simulink model "DSF_CANoe_A3"  (R2022b)
settings: configuration reference "CommonModelConfiguration" (kept outside this file)
undefined symbols (not defined in the file or in its folder): OnOff1, PsdNotPsd
libraries: canoelib x127, simulink x44
(part 2 of 3)

== system DSF_CANoe_A3/ACC//SLA ==
  Constant15 : Constant  Value=0
  Constant17 : Constant  Value=10  OutDataTypeStr=uint8
  Constant18 : Constant  OutDataTypeStr=uint8
  Constant19 : Constant  Value=0  OutDataTypeStr=uint8
  Display44 : Display
  Display48 : Display
  Signal Input3 : canoelib/CANoe I//O/Signal Input  dbName=Backbone  nodeName=DIM  msgName=DIMBackBoneSignalIPdu02  sigName=DrvrCrsCtrlWithBoostReq  editSampleTime=0  rawValue=Default  dataType=Default  dataTypeDB=uint8  hasEncoding=off
      settings: AttributesFormatString=%<sigName>  SourceProductName=Vector CANoe
  Signal Input8 : canoelib/CANoe I//O/Signal Input  dbName=Backbone  nodeName=DIM  msgName=DIMBackBoneSignalIPdu04  sigName=DrvrHmiSpdLimAdpnSts  editSampleTime=0  rawValue=Default  dataType=Default  dataTypeDB=boolean  hasEncoding=off
      settings: AttributesFormatString=%<sigName>  SourceProductName=Vector CANoe
  Signal Output15 : canoelib/CANoe I//O/Signal Output  dbName=Backbone  nodeName=ASDM  msgName=ASDMBackBoneSignalIPdu01  sigName=CnclWarnLatForAutDrv  rawValue=Default  dataType=Default  dataTypeDB=uint8  hasEncoding=off
      settings: AttributesFormatString=%<sigName>  SourceProductName=Vector CANoe
  Signal Output44 : canoelib/CANoe I//O/Signal Output  dbName=Backbone  nodeName=ASDM  msgName=ASDMBackBoneSignalIPdu07  sigName=CtryForRoadSgnInfo  rawValue=Default  dataType=Default  dataTypeDB=uint8  hasEncoding=off
      settings: AttributesFormatString=%<sigName>  SourceProductName=Vector CANoe
  Signal Output45 : canoelib/CANoe I//O/Signal Output  dbName=Backbone  nodeName=IHU  msgName=IHUBackBoneSignalIPdu03  sigName=AccAdprSpdLimActvSts  rawValue=Default  dataType=Default  dataTypeDB=boolean  hasEncoding=off
      settings: AttributesFormatString=%<sigName>  SourceProductName=Vector CANoe
  Signal Output46 : canoelib/CANoe I//O/Signal Output  dbName=Backbone  nodeName=ASDM  msgName=ASDMBackBoneSignalIPdu06  sigName=SpdLimAdpvSts  rawValue=Default  dataType=Default  dataTypeDB=uint8  hasEncoding=off
      settings: AttributesFormatString=%<sigName>  SourceProductName=Vector CANoe
  wires:
  Constant17/1 -> Signal Output44/1
  Constant15/1 -> Signal Output15/1
  Signal Input3/1 -> Display44/1
  Signal Input8/1 -> Display48/1
  Constant18/1 -> Signal Output46/1
  Constant19/1 -> Signal Output45/1

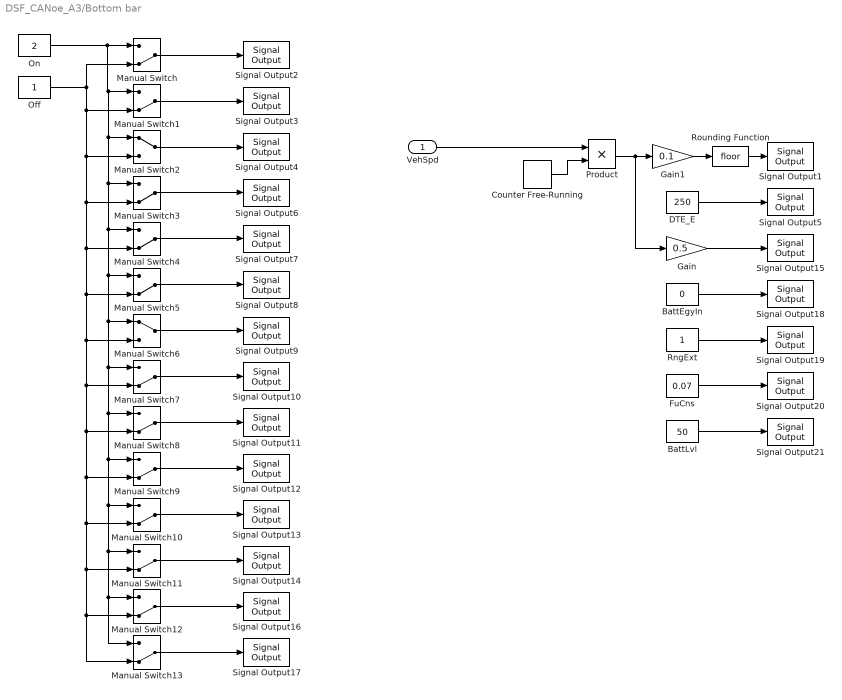
== system DSF_CANoe_A3/Bottom bar ==
  VehSpd : Inport
  BattEgyIn : Constant  Value=0  OutDataTypeStr=uint8
  BattLvl : Constant  Value=50  OutDataTypeStr=uint8
  Counter Free-Running : simulink/Sources/Counter Free-Running  NumBits=8  tsamp=-1
  DTE_E : Constant  Value=250  OutDataTypeStr=uint8
  FuCns : Constant  Value=0.07  OutDataTypeStr=uint8
  Gain : Gain  Gain=0.5
  Gain1 : Gain  Gain=0.1
  Manual Switch{,1,3..5,7..13} (12 alike) : ManualSwitch  CurrentSetting=0
  Manual Switch2 : ManualSwitch
  Manual Switch6 : ManualSwitch
  Off : Constant  OutDataTypeStr=uint8
  On : Constant  Value=2  OutDataTypeStr=uint8
  Product : Product
  RngExt : Constant  OutDataTypeStr=uint8
  Rounding Function : Rounding
  Signal Output1 : canoelib/CANoe I//O/Signal Output  dbName=Backbone  nodeName=VCU1  msgName=VDDMBackBoneSignalIpdu07  sigName=WhlRotCntrFrnt  rawValue=Default  dataType=Default  dataTypeDB=uint8  hasEncoding=off
      settings: AttributesFormatString=%<sigName>  SourceProductName=Vector CANoe
  Signal Output10 : canoelib/CANoe I//O/Signal Output  dbName=Backbone  nodeName=IHU  msgName=IHUBackBoneSignalIPdu07  sigName=SetgAndRstOfTripForDrvrSetgTripForEgyCnsAvg2  rawValue=Default  dataType=Default  dataTypeDB=uint8  hasEncoding=off
      settings: AttributesFormatString=%<sigName>  SourceProductName=Vector CANoe
  Signal Output11 : canoelib/CANoe I//O/Signal Output  dbName=Backbone  nodeName=IHU  msgName=IHUBackBoneSignalIPdu07  sigName=SetgAndRstOfTripForDrvrSetgTripForTiDrv1  rawValue=Default  dataType=Default  dataTypeDB=uint8  hasEncoding=off
      settings: AttributesFormatString=%<sigName>  SourceProductName=Vector CANoe
  Signal Output12 : canoelib/CANoe I//O/Signal Output  dbName=Backbone  nodeName=IHU  msgName=IHUBackBoneSignalIPdu07  sigName=SetgAndRstOfTripForDrvrSetgTripForTiDrv2  rawValue=Default  dataType=Default  dataTypeDB=uint8  hasEncoding=off
      settings: AttributesFormatString=%<sigName>  SourceProductName=Vector CANoe
  Signal Output13 : canoelib/CANoe I//O/Signal Output  dbName=Backbone  nodeName=IHU  msgName=IHUBackBoneSignalIPdu07  sigName=SetgAndRstOfTripForDrvrSetgTripForSpdAvg1  rawValue=Default  dataType=Default  dataTypeDB=uint8  hasEncoding=off
      settings: AttributesFormatString=%<sigName>  SourceProductName=Vector CANoe
  Signal Output14 : canoelib/CANoe I//O/Signal Output  dbName=Backbone  nodeName=IHU  msgName=IHUBackBoneSignalIPdu07  sigName=SetgAndRstOfTripForDrvrSetgTripForSpdAvg2  rawValue=Default  dataType=Default  dataTypeDB=uint8  hasEncoding=off
      settings: AttributesFormatString=%<sigName>  SourceProductName=Vector CANoe
  Signal Output15 : canoelib/CANoe I//O/Signal Output  dbName=Backbone  nodeName=VCU1  msgName=VDDMBackBoneSignalIpdu08  sigName=DispBattEgyOut  rawValue=Default  dataType=Default  dataTypeDB=uint8  hasEncoding=on
      settings: AttributesFormatString=%<sigName>  SourceProductName=Vector CANoe
  Signal Output16 : canoelib/CANoe I//O/Signal Output  dbName=Backbone  nodeName=IHU  msgName=IHUBackBoneSignalIPdu07  sigName=SetgAndRstOfTripForDrvrSetgTripWithProfID  rawValue=Default  dataType=Default  dataTypeDB=uint8  hasEncoding=off
      settings: AttributesFormatString=%<sigName>  SourceProductName=Vector CANoe
  Signal Output17 : canoelib/CANoe I//O/Signal Output  dbName=Backbone  nodeName=CEM  msgName=CEMBackBoneSignalIpdu03  sigName=ProfPenSts1  rawValue=Default  dataType=Default  dataTypeDB=uint8  hasEncoding=off
      settings: AttributesFormatString=%<sigName>  SourceProductName=Vector CANoe
  Signal Output18 : canoelib/CANoe I//O/Signal Output  dbName=Backbone  nodeName=VCU1  msgName=VDDMBackBoneSignalIpdu08  sigName=DispBattEgyIn  rawValue=Default  dataType=Default  dataTypeDB=uint8  hasEncoding=on
      settings: AttributesFormatString=%<sigName>  SourceProductName=Vector CANoe
  Signal Output19 : canoelib/CANoe I//O/Signal Output  dbName=Backbone  nodeName=VCU1  msgName=VDDMBackBoneSignalIpdu08  sigName=RngExtd  rawValue=Default  dataType=Default  dataTypeDB=uint16  hasEncoding=on
      settings: AttributesFormatString=%<sigName>  SourceProductName=Vector CANoe
  Signal Output2 : canoelib/CANoe I//O/Signal Output  dbName=Backbone  nodeName=IHU  msgName=IHUBackBoneSignalIPdu07  sigName=SetgAndRstOfTripForDrvrSetgTripForDstLong  rawValue=Default  dataType=Default  dataTypeDB=uint8  hasEncoding=off
      settings: AttributesFormatString=%<sigName>  SourceProductName=Vector CANoe
  Signal Output20 : canoelib/CANoe I//O/Signal Output  dbName=Backbone  nodeName=VCU1  msgName=VDDMBackBoneSignalIpdu09  sigName=EngFuCnsFild  rawValue=Default  dataType=Default  dataTypeDB=uint8  hasEncoding=on
      settings: AttributesFormatString=%<sigName>  SourceProductName=Vector CANoe
  Signal Output21 : canoelib/CANoe I//O/Signal Output  dbName=Backbone  nodeName=VCU1  msgName=VDDMBackBoneSignalIpdu07  sigName=DispHvBattLvlOfChrg  rawValue=Default  dataType=Default  dataTypeDB=uint16  hasEncoding=on
      settings: AttributesFormatString=%<sigName>  SourceProductName=Vector CANoe
  Signal Output3 : canoelib/CANoe I//O/Signal Output  dbName=Backbone  nodeName=IHU  msgName=IHUBackBoneSignalIPdu07  sigName=SetgAndRstOfTripForDrvrSetgTripForFuCns  rawValue=Default  dataType=Default  dataTypeDB=uint8  hasEncoding=off
      settings: AttributesFormatString=%<sigName>  SourceProductName=Vector CANoe
  Signal Output4 : canoelib/CANoe I//O/Signal Output  dbName=Backbone  nodeName=IHU  msgName=IHUBackBoneSignalIPdu07  sigName=SetgAndRstOfTripForDrvrSetgTripForDstSho1  rawValue=Default  dataType=Default  dataTypeDB=uint8  hasEncoding=off
      settings: AttributesFormatString=%<sigName>  SourceProductName=Vector CANoe
  Signal Output5 : canoelib/CANoe I//O/Signal Output  dbName=Backbone  nodeName=VCU1  msgName=VDDMBackBoneSignalIpdu08  sigName=DstEstimdToEmptyForDrvgElec  rawValue=Default  dataType=Default  dataTypeDB=uint16  hasEncoding=off
      settings: AttributesFormatString=%<sigName>  SourceProductName=Vector CANoe
  Signal Output6 : canoelib/CANoe I//O/Signal Output  dbName=Backbone  nodeName=IHU  msgName=IHUBackBoneSignalIPdu07  sigName=SetgAndRstOfTripForDrvrSetgTripForDstSho2  rawValue=Default  dataType=Default  dataTypeDB=uint8  hasEncoding=off
      settings: AttributesFormatString=%<sigName>  SourceProductName=Vector CANoe
  Signal Output7 : canoelib/CANoe I//O/Signal Output  dbName=Backbone  nodeName=IHU  msgName=IHUBackBoneSignalIPdu07  sigName=SetgAndRstOfTripForDrvrSetgTripForFuCnsAvg1  rawValue=Default  dataType=Default  dataTypeDB=uint8  hasEncoding=off
      settings: AttributesFormatString=%<sigName>  SourceProductName=Vector CANoe
  Signal Output8 : canoelib/CANoe I//O/Signal Output  dbName=Backbone  nodeName=IHU  msgName=IHUBackBoneSignalIPdu07  sigName=SetgAndRstOfTripForDrvrSetgTripForFuCnsAvg2  rawValue=Default  dataType=Default  dataTypeDB=uint8  hasEncoding=off
      settings: AttributesFormatString=%<sigName>  SourceProductName=Vector CANoe
  Signal Output9 : canoelib/CANoe I//O/Signal Output  dbName=Backbone  nodeName=IHU  msgName=IHUBackBoneSignalIPdu07  sigName=SetgAndRstOfTripForDrvrSetgTripForEgyCnsAvg1  rawValue=Default  dataType=Default  dataTypeDB=uint8  hasEncoding=off
      settings: AttributesFormatString=%<sigName>  SourceProductName=Vector CANoe
  wires:
  DTE_E/1 -> Signal Output5/1
  FuCns/1 -> Signal Output20/1
  RngExt/1 -> Signal Output19/1
  Product/1 -> Gain/1, Gain1/1
  BattEgyIn/1 -> Signal Output18/1
  Gain/1 -> Signal Output15/1
  Counter Free-Running/1 -> Product/2
  VehSpd/1 -> Product/1
  Off/1 -> Manual Switch7/2, Manual Switch8/2, Manual Switch9/2, Manual Switch13/2, Manual Switch12/2, Manual Switch11/2, Manual Switch10/2, Manual Switch6/2, Manual Switch5/2, Manual Switch4/2, Manual Switch3/2, Manual Switch2/2, Manual Switch1/2, Manual Switch/2
  Manual Switch/1 -> Signal Output2/1
  On/1 -> Manual Switch2/1, Manual Switch11/1, Manual Switch13/1, Manual Switch12/1, Manual Switch10/1, Manual Switch9/1, Manual Switch8/1, Manual Switch7/1, Manual Switch6/1, Manual Switch5/1, Manual Switch4/1, Manual Switch3/1, Manual Switch1/1, Manual Switch/1
  Manual Switch1/1 -> Signal Output3/1
  Manual Switch2/1 -> Signal Output4/1
  Manual Switch3/1 -> Signal Output6/1
  Manual Switch4/1 -> Signal Output7/1
  Manual Switch5/1 -> Signal Output8/1
  Manual Switch6/1 -> Signal Output9/1
  Manual Switch10/1 -> Signal Output13/1
  Manual Switch13/1 -> Signal Output17/1
  Manual Switch12/1 -> Signal Output16/1
  Manual Switch11/1 -> Signal Output14/1
  Manual Switch9/1 -> Signal Output12/1
  Manual Switch8/1 -> Signal Output11/1
  Manual Switch7/1 -> Signal Output10/1
  BattLvl/1 -> Signal Output21/1
  Gain1/1 -> Rounding Function/1
  Rounding Function/1 -> Signal Output1/1

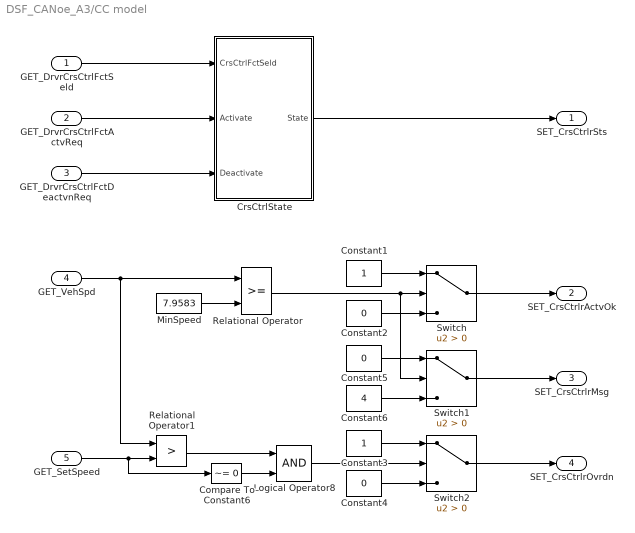
== system DSF_CANoe_A3/CC model ==
  GET_DrvrCrsCtrlFctSeld : Inport
  GET_DrvrCrsCtrlFctActvReq : Inport  Port=2
  GET_DrvrCrsCtrlFctDeactvnReq : Inport  Port=3
  GET_VehSpd : Inport  Port=4
  GET_SetSpeed : Inport  Port=5
  Compare To Constant6 : simulink/Logic and Bit Operations/Compare To Constant  relop=~=  const=0  OutDataTypeStr=boolean
  Constant1 : Constant  OutDataTypeStr=uint8
  Constant2 : Constant  Value=0  OutDataTypeStr=uint8
  Constant3 : Constant  OutDataTypeStr=uint8
  Constant4 : Constant  Value=0  OutDataTypeStr=uint8
  Constant5 : Constant  Value=0  OutDataTypeStr=uint8
  Constant6 : Constant  Value=4  OutDataTypeStr=uint8
  CrsCtrlState : Stateflow chart  TreatAsAtomicUnit=on
  Logical Operator8 : Logic  AllPortsSameDT=off  OutDataTypeStr=boolean
  MinSpeed : Constant  Value=7.9583
  Relational Operator : RelationalOperator  OutDataTypeStr=boolean  RndMeth=Simplest  InputSameDT=off
  Relational Operator1 : RelationalOperator  Operator=>  OutDataTypeStr=boolean  RndMeth=Simplest  InputSameDT=off
  Switch : Switch  Criteria=u2 > Threshold  SaturateOnIntegerOverflow=off  InputSameDT=off
  Switch1 : Switch  Criteria=u2 > Threshold  SaturateOnIntegerOverflow=off  InputSameDT=off
  Switch2 : Switch  Criteria=u2 > Threshold  SaturateOnIntegerOverflow=off  InputSameDT=off
  SET_CrsCtrlrSts : Outport
  SET_CrsCtrlrActvOk : Outport  Port=2
  SET_CrsCtrlrMsg : Outport  Port=3
  SET_CrsCtrlrOvrdn : Outport  Port=4
  wires:
  Constant1/1 -> Switch/1
  Relational Operator/1 -> Switch1/2, Switch/2
  GET_VehSpd/1 -> Relational Operator1/1, Relational Operator/1
  Switch/1 -> SET_CrsCtrlrActvOk/1
  Constant2/1 -> Switch/3
  Switch1/1 -> SET_CrsCtrlrMsg/1
  Constant5/1 -> Switch1/1
  Constant6/1 -> Switch1/3
  Switch2/1 -> SET_CrsCtrlrOvrdn/1
  Constant3/1 -> Switch2/1
  Constant4/1 -> Switch2/3
  CrsCtrlState/1(State) -> SET_CrsCtrlrSts/1
  GET_DrvrCrsCtrlFctActvReq/1 -> CrsCtrlState/2(Activate)
  GET_DrvrCrsCtrlFctSeld/1 -> CrsCtrlState/1(CrsCtrlFctSeld)
  GET_DrvrCrsCtrlFctDeactvnReq/1 -> CrsCtrlState/3(Deactivate)
  MinSpeed/1 -> Relational Operator/2
  Relational Operator1/1 -> Logical Operator8/1
  Compare To Constant6/1 -> Logical Operator8/2
  GET_SetSpeed/1 -> Compare To Constant6/1, Relational Operator1/2
  Logical Operator8/1 -> Switch2/2

== system DSF_CANoe_A3/CSA model ==
  Compare To Constant1 : simulink/Logic and Bit Operations/Compare To Constant  relop=<  const=3  OutDataTypeStr=boolean
  Compare To Constant2 : simulink/Logic and Bit Operations/Compare To Constant  relop=~=  const=0  OutDataTypeStr=boolean
  Compare To Constant3 : simulink/Logic and Bit Operations/Compare To Constant  relop=>  const=2  OutDataTypeStr=boolean
  Constant14 : Constant  Value=0  OutDataTypeStr=uint8
  multiply : Product
  multiply1 : Product
  SET_CrvtSpdAdpvSts : Outport
  SET_DirOfCrvtSpdCtrl : Outport  Port=2
  SET_SpdAdjmtEve : Outport  Port=3
  wires:
  Compare To Constant2/1 -> SET_CrvtSpdAdpvSts/1
  Constant14/1 -> Compare To Constant3/1, multiply1/1, Compare To Constant1/1, multiply/1, Compare To Constant2/1
  Compare To Constant1/1 -> multiply/2
  multiply/1 -> SET_DirOfCrvtSpdCtrl/1
  multiply1/1 -> SET_SpdAdjmtEve/1
  Compare To Constant3/1 -> multiply1/2

== system DSF_CANoe_A3/Common ==
  Constant : Constant  Value=13
  Constant1 : Constant
  Constant2 : Constant  Value=0
  Constant28 : Constant  Value=0
  Constant30 : Constant  OutDataTypeStr=uint8
  Signal Output : canoelib/CANoe I//O/Signal Output  dbName=Backbone  nodeName=CEM  msgName=CEMBackBoneSignalIpdu01  sigName=UsgModSts  rawValue=Default  dataType=Default  dataTypeDB=uint8  hasEncoding=off
      settings: AttributesFormatString=%<sigName>  SourceProductName=Vector CANoe
  Signal Output1 : canoelib/CANoe I//O/Signal Output  dbName=Backbone  nodeName=CEM  msgName=CEMBackBoneSignalIpdu01  sigName=CarModSts1  rawValue=Default  dataType=Default  dataTypeDB=uint8  hasEncoding=off
      settings: AttributesFormatString=%<sigName>  SourceProductName=Vector CANoe
  Signal Output18 : canoelib/CANoe I//O/Signal Output  dbName=Backbone  nodeName=IHU  msgName=IHUBackBoneSignalIPdu02  sigName=SpdUnit  rawValue=Default  dataType=Default  dataTypeDB=uint8  hasEncoding=off
      settings: AttributesFormatString=%<sigName>  SourceProductName=Vector CANoe
  Signal Output19 : canoelib/CANoe I//O/Signal Output  dbName=Backbone  nodeName=ASDM  msgName=ASDMBackBoneSignalIPdu07  sigName=SpdLimUnit  rawValue=Default  dataType=Default  dataTypeDB=boolean  hasEncoding=off
      settings: AttributesFormatString=%<sigName>  SourceProductName=Vector CANoe
  Signal Output39 : canoelib/CANoe I//O/Signal Output  dbName=Backbone  nodeName=VCU1  msgName=VDDMBackBoneSignalIPdu19  sigName=HmiAutnmsStsHmiAutnmsSts  rawValue=Default  dataType=Default  dataTypeDB=uint8  hasEncoding=off
      settings: AttributesFormatString=%<sigName>  SourceProductName=Vector CANoe
  Signal Output5 : canoelib/CANoe I//O/Signal Output  dbName=Backbone  nodeName=IHU  msgName=IHUBackBoneSignalIPdu07  sigName=UsrSeldDrvrSpprtFct  rawValue=Default  dataType=Default  dataTypeDB=uint8  hasEncoding=off
      settings: AttributesFormatString=%<sigName>  SourceProductName=Vector CANoe
  SpeedUnit : Constant  Value=0
  wires:
  Constant1/1 -> Signal Output5/1
  Constant28/1 -> Signal Output19/1
  Constant2/1 -> Signal Output1/1
  Constant30/1 -> Signal Output39/1
  Constant/1 -> Signal Output/1
  SpeedUnit/1 -> Signal Output18/1

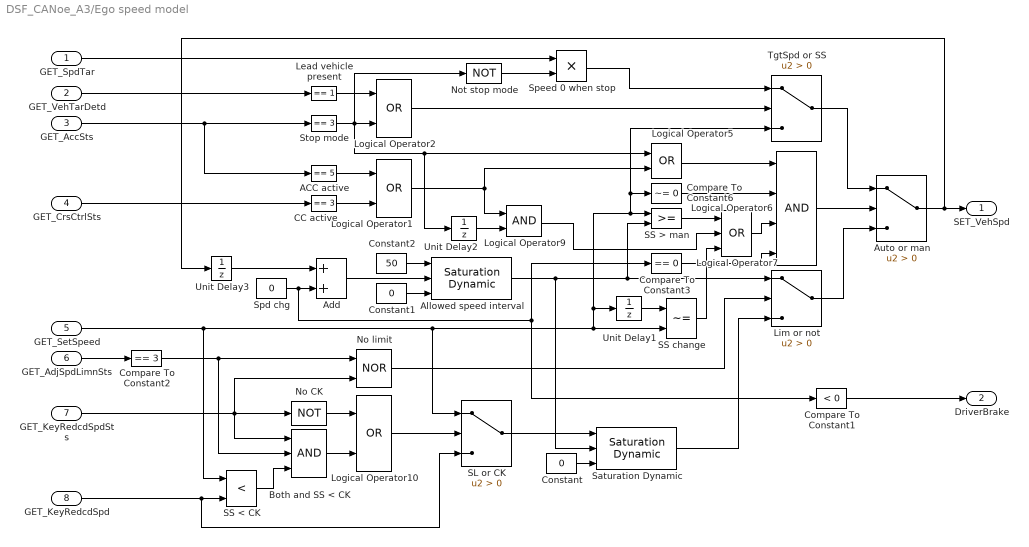
== system DSF_CANoe_A3/Ego speed model ==
  GET_SpdTar : Inport
  GET_VehTarDetd : Inport  Port=2
  GET_AccSts : Inport  Port=3
  GET_CrsCtrlSts : Inport  Port=4
  GET_SetSpeed : Inport  Port=5
  GET_AdjSpdLimnSts : Inport  Port=6
  GET_KeyRedcdSpdSts : Inport  Port=7
  GET_KeyRedcdSpd : Inport  Port=8
  ACC active : simulink/Logic and Bit Operations/Compare To Constant  relop===  const=5  OutDataTypeStr=boolean
  Add : Sum
  Allowed speed interval : simulink/Discontinuities/Saturation Dynamic  OutMin=0  OutMax=[]  OutDataTypeStr=Inherit: Same as second input  OutDataType=fixdt(1, 16)  OutScaling=2^-10  DoSatur=off
  Auto or man : Switch  Criteria=u2 > Threshold  SaturateOnIntegerOverflow=off  InputSameDT=off
  Both and SS < CK : Logic  Inputs=3  AllPortsSameDT=off  OutDataTypeStr=boolean
  CC active : simulink/Logic and Bit Operations/Compare To Constant  relop===  const=3  OutDataTypeStr=boolean
  Compare To Constant1 : simulink/Logic and Bit Operations/Compare To Constant  relop=<  const=0  OutDataTypeStr=boolean
  Compare To Constant2 : simulink/Logic and Bit Operations/Compare To Constant  relop===  const=3  OutDataTypeStr=boolean
  Compare To Constant3 : simulink/Logic and Bit Operations/Compare To Constant  relop===  const=0  OutDataTypeStr=boolean
  Compare To Constant6 : simulink/Logic and Bit Operations/Compare To Constant  relop=~=  const=0  OutDataTypeStr=boolean
  Constant : Constant  Value=0
  Constant1 : Constant  Value=0
  Constant2 : Constant  Value=50
  Lead vehicle present : simulink/Logic and Bit Operations/Compare To Constant  relop===  const=1  OutDataTypeStr=boolean
  Lim or not : Switch  Criteria=u2 > Threshold  SaturateOnIntegerOverflow=off  InputSameDT=off
  Logical Operator{1..2,5,10} (4 alike) : Logic  Operator=OR  AllPortsSameDT=off  OutDataTypeStr=boolean
  Logical Operator6 : Logic  Inputs=4  AllPortsSameDT=off  OutDataTypeStr=boolean
  Logical Operator7 : Logic  Operator=OR  Inputs=3  AllPortsSameDT=off  OutDataTypeStr=boolean
  Logical Operator9 : Logic  AllPortsSameDT=off  OutDataTypeStr=boolean
  No CK : Logic  Operator=NOT  AllPortsSameDT=off  OutDataTypeStr=boolean
  No limit : Logic  Operator=NOR  AllPortsSameDT=off  OutDataTypeStr=boolean
  Not stop mode : Logic  Operator=NOT  AllPortsSameDT=off  OutDataTypeStr=boolean
  SL or CK : Switch  Criteria=u2 > Threshold  SaturateOnIntegerOverflow=off  InputSameDT=off
  SS < CK : RelationalOperator  Operator=<  OutDataTypeStr=boolean  RndMeth=Simplest  InputSameDT=off
  SS > man : RelationalOperator  OutDataTypeStr=boolean  RndMeth=Simplest  InputSameDT=off
  SS change : RelationalOperator  Operator=~=  OutDataTypeStr=boolean  RndMeth=Simplest  InputSameDT=off
  Saturation Dynamic : simulink/Discontinuities/Saturation Dynamic  OutMin=0  OutMax=[]  OutDataTypeStr=Inherit: Same as second input  OutDataType=fixdt(1, 16)  OutScaling=2^-10  DoSatur=off
  Spd chg : Constant  Value=0  OutDataTypeStr=double
  Speed 0 when stop : Product
  Stop mode : simulink/Logic and Bit Operations/Compare To Constant  relop===  const=3  OutDataTypeStr=boolean
  TgtSpd or SS : Switch  Criteria=u2 > Threshold  SaturateOnIntegerOverflow=off  InputSameDT=off
  Unit Delay1 : UnitDelay  InitialCondition=100  SampleTime=-1  HasFrameUpgradeWarning=on
  Unit Delay2 : UnitDelay  InitialCondition=1  SampleTime=-1  HasFrameUpgradeWarning=on
  Unit Delay3 : UnitDelay  InitialCondition=12  SampleTime=-1  HasFrameUpgradeWarning=on
  SET_VehSpd : Outport
  DriverBrake : Outport  Port=2
  wires:
  CC active/1 -> Logical Operator1/2
  Allowed speed interval/1 -> SS > man/2, Lim or not/1, Saturation Dynamic/2
  Auto or man/1 -> Unit Delay3/1, SET_VehSpd/1
  Lead vehicle present/1 -> Logical Operator2/1
  GET_VehTarDetd/1 -> Lead vehicle present/1
  GET_AccSts/1 -> ACC active/1, Stop mode/1
  GET_AdjSpdLimnSts/1 -> Compare To Constant2/1
  Saturation Dynamic/1 -> Lim or not/3
  Constant/1 -> Saturation Dynamic/3
  GET_KeyRedcdSpdSts/1 -> Both and SS < CK/1, No CK/1, No limit/2
  GET_KeyRedcdSpd/1 -> SL or CK/3, SS < CK/2
  Logical Operator2/1 -> TgtSpd or SS/2
  SL or CK/1 -> Saturation Dynamic/1
  Compare To Constant2/1 -> Both and SS < CK/2, No limit/1
  No limit/1 -> Lim or not/2
  Lim or not/1 -> Auto or man/3
  Both and SS < CK/1 -> Logical Operator10/2
  Logical Operator10/1 -> SL or CK/2
  SS < CK/1 -> Both and SS < CK/3
  No CK/1 -> Logical Operator10/1
  TgtSpd or SS/1 -> Auto or man/1
  Speed 0 when stop/1 -> TgtSpd or SS/1
  Not stop mode/1 -> Speed 0 when stop/2
  ACC active/1 -> Logical Operator1/1
  Logical Operator1/1 -> Logical Operator9/1, Logical Operator5/2
  Stop mode/1 -> Unit Delay2/1, Logical Operator5/1, Logical Operator2/2, Not stop mode/1
  Logical Operator5/1 -> Logical Operator6/1
  Unit Delay3/1 -> Add/1
  Spd chg/1 -> Compare To Constant1/1, Compare To Constant3/1, Add/2
  Add/1 -> Allowed speed interval/2
  Constant1/1 -> Allowed speed interval/3
  Constant2/1 -> Allowed speed interval/1
  SS > man/1 -> Logical Operator7/1
  Compare To Constant6/1 -> Logical Operator6/2
  Unit Delay1/1 -> SS change/1
  Logical Operator6/1 -> Auto or man/2
  SS change/1 -> Logical Operator7/3
  Logical Operator7/1 -> Logical Operator6/3
  Compare To Constant1/1 -> DriverBrake/1
  Logical Operator9/1 -> Logical Operator7/2
  Unit Delay2/1 -> Logical Operator9/2
  GET_CrsCtrlSts/1 -> CC active/1
  GET_SetSpeed/1 -> SL or CK/1, SS change/2, Unit Delay1/1, TgtSpd or SS/3, Compare To Constant6/1, SS > man/1, SS < CK/1
  GET_SpdTar/1 -> Speed 0 when stop/1
  Compare To Constant3/1 -> Logical Operator6/4

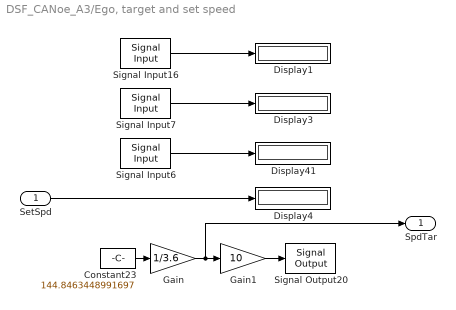
== system DSF_CANoe_A3/Ego, target and set speed ==
  SetSpd : Inport
  Constant23 : Constant  Value=144.8463448991697  OutDataTypeStr=double
  Display{1,3..4,41} (4 alike) : Display
  Gain : Gain  Gain=1/3.6  OutDataTypeStr=double
  Gain1 : Gain  Gain=10  OutDataTypeStr=uint16
  Signal Input16 : canoelib/CANoe I//O/Signal Input  dbName=Backbone  nodeName=DIM  msgName=DIMBackBoneSignalIPdu01  sigName=VehSpdIndcdVal  editSampleTime=0  rawValue=Default  dataType=Default  dataTypeDB=uint16  hasEncoding=off
      settings: AttributesFormatString=%<sigName>  SourceProductName=Vector CANoe
  Signal Input6 : canoelib/CANoe I//O/Signal Input  dbName=Backbone  nodeName=DIM  msgName=DIMBackBoneSignalIPdu04  sigName=SetSpdForDispToDrvrVal  editSampleTime=0  rawValue=Default  dataType=Default  dataTypeDB=uint16  hasEncoding=off
      settings: AttributesFormatString=%<sigName>  SourceProductName=Vector CANoe
  Signal Input7 : canoelib/CANoe I//O/Signal Input  dbName=Backbone  nodeName=DIM  msgName=DIMBackBoneSignalIPdu04  sigName=SetSpdSts  editSampleTime=0  rawValue=Default  dataType=Default  dataTypeDB=uint8  hasEncoding=off
      settings: AttributesFormatString=%<sigName>  SourceProductName=Vector CANoe
  Signal Output20 : canoelib/CANoe I//O/Signal Output  dbName=Backbone  nodeName=ASDM  msgName=ASDMBackBoneSignalIPdu06  sigName=SpdTarForDisp  rawValue=Raw value  dataType=inherited  dataTypeDB=uint16  hasEncoding=on
      settings: AttributesFormatString=%<sigName>  SourceProductName=Vector CANoe
  SpdTar : Outport
  wires:
  Gain1/1 -> Signal Output20/1
  Signal Input6/1 -> Display41/1
  Signal Input7/1 -> Display3/1
  SetSpd/1 -> Display4/1
  Gain/1 -> SpdTar/1, Gain1/1
  Constant23/1 -> Gain/1
  Signal Input16/1 -> Display1/1

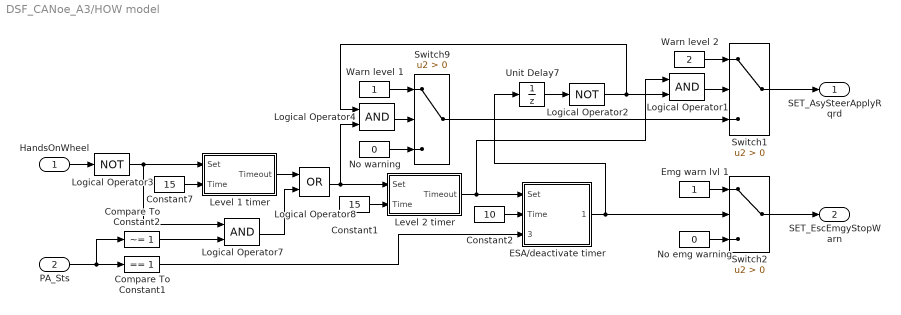
== system DSF_CANoe_A3/HOW model ==
  HandsOnWheel : Inport
  PA_Sts : Inport  Port=2
  Compare To Constant1 : simulink/Logic and Bit Operations/Compare To Constant  relop===  const=1  OutDataTypeStr=boolean
  Compare To Constant2 : simulink/Logic and Bit Operations/Compare To Constant  relop=~=  const=1  OutDataTypeStr=boolean
  Constant1 : Constant  Value=15
  Constant2 : Constant  Value=10
  Constant7 : Constant  Value=15
  ESA/deactivate timer : Stateflow chart  TreatAsAtomicUnit=on
  Emg warn lvl 1 : Constant
  Level 1 timer : Stateflow chart  TreatAsAtomicUnit=on
  Level 2 timer : Stateflow chart  TreatAsAtomicUnit=on
  Logical Operator1 : Logic  AllPortsSameDT=off  OutDataTypeStr=boolean
  Logical Operator2 : Logic  Operator=NOT  AllPortsSameDT=off  OutDataTypeStr=boolean
  Logical Operator3 : Logic  Operator=NOT  AllPortsSameDT=off  OutDataTypeStr=boolean
  Logical Operator4 : Logic  AllPortsSameDT=off  OutDataTypeStr=boolean
  Logical Operator7 : Logic  AllPortsSameDT=off  OutDataTypeStr=boolean
  Logical Operator8 : Logic  Operator=OR  AllPortsSameDT=off  OutDataTypeStr=boolean
  No emg warning : Constant  Value=0
  No warning : Constant  Value=0
  Switch1 : Switch  Criteria=u2 > Threshold  SaturateOnIntegerOverflow=off  InputSameDT=off
  Switch2 : Switch  Criteria=u2 > Threshold  SaturateOnIntegerOverflow=off  InputSameDT=off
  Switch9 : Switch  Criteria=u2 > Threshold  SaturateOnIntegerOverflow=off  InputSameDT=off
  Unit Delay7 : UnitDelay  InitialCondition=1  SampleTime=-1  HasFrameUpgradeWarning=on
  Warn level 1 : Constant
  Warn level 2 : Constant  Value=2
  SET_AsySteerApplyRqrd : Outport
  SET_EscEmgyStopWarn : Outport  Port=2
  wires:
  Constant7/1 -> Level 1 timer/2(Time)
  HandsOnWheel/1 -> Logical Operator3/1
  Constant1/1 -> Level 2 timer/2(Time)
  No warning/1 -> Switch9/3
  Warn level 1/1 -> Switch9/1
  Switch9/1 -> Switch1/3
  Warn level 2/1 -> Switch1/1
  Switch1/1 -> SET_AsySteerApplyRqrd/1
  Level 2 timer/1(Timeout) -> ESA/deactivate timer/1(Set), Logical Operator1/1
  Constant2/1 -> ESA/deactivate timer/2(Time)
  No emg warning/1 -> Switch2/3
  Switch2/1 -> SET_EscEmgyStopWarn/1
  Emg warn lvl 1/1 -> Switch2/1
  Logical Operator3/1 -> Logical Operator7/1, Level 1 timer/1(Set)
  Logical Operator1/1 -> Switch1/2
  Logical Operator2/1 -> Logical Operator4/1, Logical Operator1/2
  Unit Delay7/1 -> Logical Operator2/1
  Logical Operator4/1 -> Switch9/2
  Compare To Constant2/1 -> Logical Operator7/2
  ESA/deactivate timer/1(Timeout) -> Switch2/2, Unit Delay7/1
  Level 1 timer/1(Timeout) -> Logical Operator8/1
  Logical Operator7/1 -> Logical Operator8/2
  Logical Operator8/1 -> Logical Operator4/2, Level 2 timer/1(Set)
  PA_Sts/1 -> Compare To Constant1/1, Compare To Constant2/1
  Compare To Constant1/1 -> ESA/deactivate timer/3(PA_act)

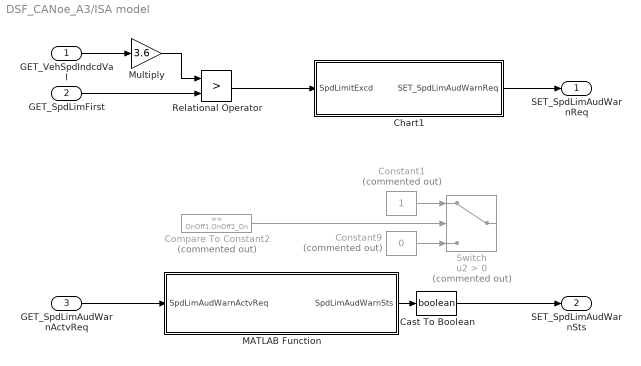
== system DSF_CANoe_A3/ISA model ==
  GET_VehSpdIndcdVal : Inport
  GET_SpdLimFirst : Inport  Port=2
  GET_SpdLimAudWarnActvReq : Inport  Port=3  OutDataTypeStr=boolean
  Cast To Boolean : DataTypeConversion  OutDataTypeStr=boolean  SaturateOnIntegerOverflow=off  RndMeth=Floor
  Chart1 : Stateflow chart  TreatAsAtomicUnit=on
  Compare To Constant2 : simulink/Logic and Bit Operations/Compare To Constant  Commented=on  relop===  const=OnOff1.OnOff1_On  OutDataTypeStr=boolean
  Constant1 : Constant  Commented=on  OutDataTypeStr=boolean
  Constant9 : Constant  Commented=on  Value=0  OutDataTypeStr=boolean
  MATLAB Function : MATLAB Function  TreatAsAtomicUnit=on
  Multiply : Gain  Gain=3.6
  Relational Operator : RelationalOperator  Operator=>  OutDataTypeStr=boolean  RndMeth=Simplest  InputSameDT=off
  Switch : Switch  Commented=on  Criteria=u2 > Threshold  SaturateOnIntegerOverflow=off  InputSameDT=off
  SET_SpdLimAudWarnReq : Outport
  SET_SpdLimAudWarnSts : Outport  Port=2
  wires:
  Relational Operator/1 -> Chart1/1(SpdLimitExcd)
  GET_SpdLimFirst/1 -> Relational Operator/2
  Chart1/1(SET_SpdLimAudWarnReq) -> SET_SpdLimAudWarnReq/1
  Compare To Constant2/1 -> Switch/2
  Constant1/1 -> Switch/1
  Constant9/1 -> Switch/3
  MATLAB Function/1(SpdLimAudWarnSts) -> Cast To Boolean/1
  GET_SpdLimAudWarnActvReq/1 -> MATLAB Function/1(SpdLimAudWarnActvReq)
  Cast To Boolean/1 -> SET_SpdLimAudWarnSts/1
  GET_VehSpdIndcdVal/1 -> Multiply/1
  Multiply/1 -> Relational Operator/1

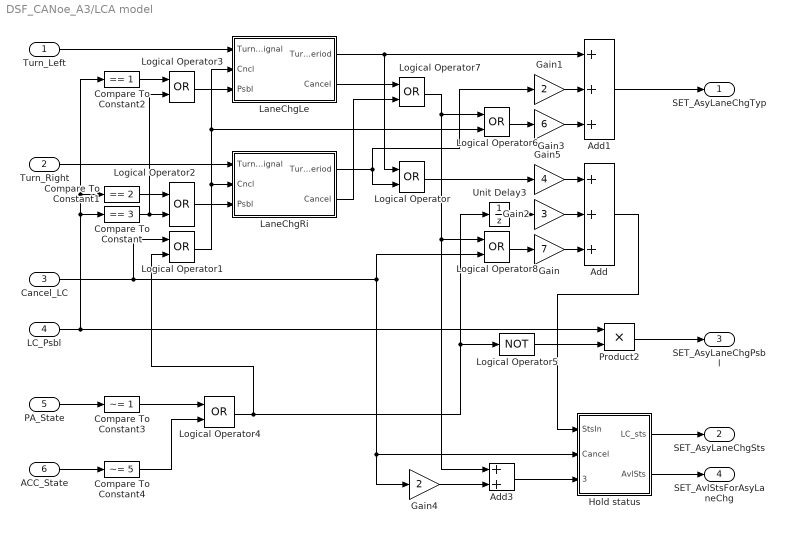
== system DSF_CANoe_A3/LCA model ==
  Turn_Left : Inport
  Turn_Right : Inport  Port=2
  Cancel_LC : Inport  Port=3
  LC_Psbl : Inport  Port=4
  PA_State : Inport  Port=5
  ACC_State : Inport  Port=6
  Add : Sum  Inputs=+++
  Add1 : Sum  Inputs=+++
  Add3 : Sum
  Compare To Constant : simulink/Logic and Bit Operations/Compare To Constant  relop===  const=3  OutDataTypeStr=boolean
  Compare To Constant1 : simulink/Logic and Bit Operations/Compare To Constant  relop===  const=2  OutDataTypeStr=boolean
  Compare To Constant2 : simulink/Logic and Bit Operations/Compare To Constant  relop===  const=1  OutDataTypeStr=boolean
  Compare To Constant3 : simulink/Logic and Bit Operations/Compare To Constant  relop=~=  const=1  OutDataTypeStr=boolean
  Compare To Constant4 : simulink/Logic and Bit Operations/Compare To Constant  relop=~=  const=5  OutDataTypeStr=boolean
  Gain : Gain  Gain=7  OutDataTypeStr=uint8
  Gain1 : Gain  Gain=2  OutDataTypeStr=uint8
  Gain2 : Gain  Gain=3  OutDataTypeStr=uint8
  Gain3 : Gain  Gain=6  OutDataTypeStr=uint8
  Gain4 : Gain  Gain=2  OutDataTypeStr=uint8
  Gain5 : Gain  Gain=4  OutDataTypeStr=uint8
  Hold status : Stateflow chart  TreatAsAtomicUnit=on
      settings: PortSchema="{\"entries\":[{\"content\":{\"sides\":[{\"content\":{\"connectorIds\":[\"In1\",\"In2\",\"In3\"]},\"type\":\"ConnectorPlacement.EquallySpacedRectSide\",\"uuid\":\"a87ca77b-bf2e-41ea-800c-013664d6dc40\"},{\"content\":{\"connectorIds\":[\"Out2\",\"Out1\"],\"side\":\"RIGHT\"},\"type\":\"ConnectorPlacement.EquallySpacedRectSide\",\"uuid\":\"d37128e6-dd28-43be-9ab0-e23ef9c90c45\"},{\"content\":{\"connectorIds\":[],\"side\":\"TOP\"},\"type\":\"ConnectorPlacement.EquallySpacedRectSide\",\"uuid\":\"b070bec6-d3f7-4036-8dc0-3a15dab46598\"}]},\"type\":\"ConnectorPlacement.EquallySpacedConnector\",\"uuid\":\"f07aa533-0e27-4703-9126-1d110d006581\"}],\"packageUris\":[\"http://schema.mathworks.com/mf0/Connector/R2020b\"],\"version\":\"1.0\"}"
  LaneChgLe : Stateflow chart  TreatAsAtomicUnit=on
  LaneChgRi : Stateflow chart  TreatAsAtomicUnit=on
  Logical Operator{,1..4,6..8} (8 alike) : Logic  Operator=OR  AllPortsSameDT=off  OutDataTypeStr=boolean
  Logical Operator5 : Logic  Operator=NOT  AllPortsSameDT=off  OutDataTypeStr=boolean
  Product2 : Product  OutDataTypeStr=uint8
  Unit Delay3 : UnitDelay  SampleTime=-1  HasFrameUpgradeWarning=on
  SET_AsyLaneChgTyp : Outport
  SET_AsyLaneChgSts : Outport  Port=2
  SET_AsyLaneChgPsbl : Outport  Port=3
  SET_AvlStsForAsyLaneChg : Outport  Port=4
  wires:
  Add/1 -> Hold status/1(StsIn)
  Add1/1 -> SET_AsyLaneChgTyp/1
  Add3/1 -> Hold status/3(AvlStsIn)
  Compare To Constant2/1 -> Logical Operator3/1
  Compare To Constant4/1 -> Logical Operator4/2
  LaneChgRi/2(Cancel) -> Logical Operator7/2
  LaneChgLe/2(Cancel) -> Logical Operator7/1
  Product2/1 -> SET_AsyLaneChgPsbl/1
  Gain1/1 -> Add1/2
  Logical Operator7/1 -> Logical Operator8/1, Add3/1, Logical Operator6/1
  Gain3/1 -> Add1/3
  Logical Operator/1 -> Gain5/1
  Compare To Constant/1 -> Logical Operator3/2, Logical Operator2/2
  Logical Operator5/1 -> Product2/2
  Logical Operator3/1 -> LaneChgLe/3(Psbl)
  Gain/1 -> Add/3
  PA_State/1 -> Compare To Constant3/1
  Gain4/1 -> Add3/2
  Logical Operator1/1 -> LaneChgRi/2(Cncl), LaneChgLe/2(Cncl), Logical Operator6/2
  Compare To Constant3/1 -> Logical Operator4/1
  Logical Operator2/1 -> LaneChgRi/3(Psbl)
  Turn_Left/1 -> LaneChgLe/1(TurnSignal)
  Logical Operator6/1 -> Gain3/1
  Compare To Constant1/1 -> Logical Operator2/1
  Gain2/1 -> Add/2
  LaneChgRi/1(TurnPeriod) -> Gain1/1, Logical Operator/2
  Logical Operator8/1 -> Gain/1
  Cancel_LC/1 -> Logical Operator1/1, Logical Operator8/2, Gain4/1, Hold status/2(Cancel)
  LaneChgLe/1(TurnPeriod) -> Logical Operator/1, Add1/1
  LC_Psbl/1 -> Product2/1, Compare To Constant2/1, Compare To Constant1/1, Compare To Constant/1
  ACC_State/1 -> Compare To Constant4/1
  Turn_Right/1 -> LaneChgRi/1(TurnSignal)
  Gain5/1 -> Add/1
  Logical Operator4/1 -> Logical Operator1/2, Unit Delay3/1, Logical Operator5/1
  Unit Delay3/1 -> Gain2/1
  Hold status/1(AvlSts) -> SET_AvlStsForAsyLaneChg/1
  Hold status/2(LC_sts) -> SET_AsyLaneChgSts/1

== system DSF_CANoe_A3/LKA ==
  LaneDetSts : Inport
  Constant31 : Constant  OutDataTypeStr=uint8
  Constant32 : Constant  OutDataTypeStr=uint8
  Constant34 : Constant  Value=0  OutDataTypeStr=uint8
  Constant35 : Constant  Value=0  OutDataTypeStr=uint8
  No lanes always : Constant  Value=0
  Signal Output55 : canoelib/CANoe I//O/Signal Output  dbName=Backbone  nodeName=IHU  msgName=IHUBackBoneSignalIPdu02  sigName=LaneKeepAidActvSts  rawValue=Default  dataType=Default  dataTypeDB=boolean  hasEncoding=off
      settings: AttributesFormatString=%<sigName>  SourceProductName=Vector CANoe
  Signal Output56 : canoelib/CANoe I//O/Signal Output  dbName=Backbone  nodeName=ASDM  msgName=ASDMBackBoneSignalIPdu07  sigName=LaneKeepAidSts  rawValue=Default  dataType=Default  dataTypeDB=uint8  hasEncoding=off
      settings: AttributesFormatString=%<sigName>  SourceProductName=Vector CANoe
  Signal Output57 : canoelib/CANoe I//O/Signal Output  dbName=Backbone  nodeName=ASDM  msgName=ASDMBackBoneSignalIPdu06  sigName=LaneDetnStsForLaneKeepAid  rawValue=Default  dataType=Default  dataTypeDB=uint8  hasEncoding=off
      settings: AttributesFormatString=%<sigName>  SourceProductName=Vector CANoe
  Signal Output58 : canoelib/CANoe I//O/Signal Output  dbName=Backbone  nodeName=IHU  msgName=IHUBackBoneSignalIPdu02  sigName=LaneChgWarnActvSts  rawValue=Default  dataType=Default  dataTypeDB=boolean  hasEncoding=off
      settings: AttributesFormatString=%<sigName>  SourceProductName=Vector CANoe
  Signal Output59 : canoelib/CANoe I//O/Signal Output  dbName=Backbone  nodeName=ASDM  msgName=ASDMBackBoneSignalIPdu06  sigName=SteerIntvSts  rawValue=Default  dataType=Default  dataTypeDB=uint8  hasEncoding=off
      settings: AttributesFormatString=%<sigName>  SourceProductName=Vector CANoe
  Terminator : Terminator
  wires:
  Constant32/1 -> Signal Output56/1
  Constant34/1 -> Signal Output58/1
  Constant35/1 -> Signal Output59/1
  Constant31/1 -> Signal Output55/1
  LaneDetSts/1 -> Terminator/1
  No lanes always/1 -> Signal Output57/1

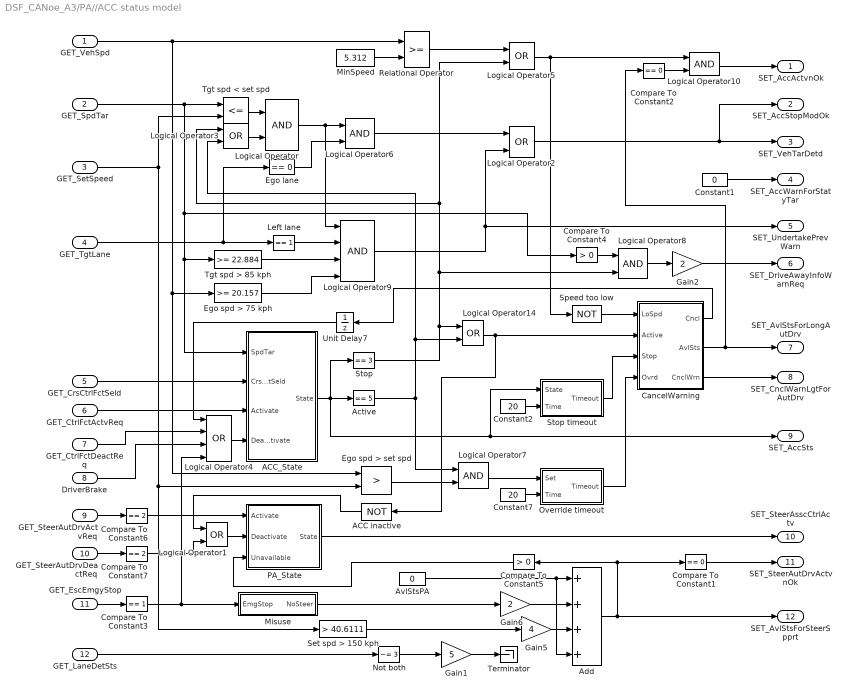
== system DSF_CANoe_A3/PA//ACC status model ==
  GET_VehSpd : Inport
  GET_SpdTar : Inport  Port=2
  GET_SetSpeed : Inport  Port=3
  GET_TgtLane : Inport  Port=4
  GET_CrsCtrlFctSeld : Inport  Port=5
  GET_CtrlFctActvReq : Inport  Port=6
  GET_CtrlFctDeactReq : Inport  Port=7
  DriverBrake : Inport  Port=8
  GET_SteerAutDrvActvReq : Inport  Port=9
  GET_SteerAutDrvDeactReq : Inport  Port=10
  GET_EscEmgyStop : Inport  Port=11
  GET_LaneDetSts : Inport  Port=12
  ACC inactive : Logic  Operator=NOT  AllPortsSameDT=off  OutDataTypeStr=boolean
  ACC_State : Stateflow chart  TreatAsAtomicUnit=on
  Active : simulink/Logic and Bit Operations/Compare To Constant  relop===  const=5  OutDataTypeStr=boolean
  Add : Sum  Inputs=++++
  AvlStsPA : Constant  Value=0
  CancelWarning : Subsystem
  Compare To Constant1 : simulink/Logic and Bit Operations/Compare To Constant  relop===  const=0  OutDataTypeStr=boolean
  Compare To Constant2 : simulink/Logic and Bit Operations/Compare To Constant  relop===  const=0  OutDataTypeStr=boolean
  Compare To Constant3 : simulink/Logic and Bit Operations/Compare To Constant  relop===  const=1  OutDataTypeStr=boolean
  Compare To Constant4 : simulink/Logic and Bit Operations/Compare To Constant  relop=>  const=0  OutDataTypeStr=boolean
  Compare To Constant5 : simulink/Logic and Bit Operations/Compare To Constant  relop=>  const=0  OutDataTypeStr=boolean
  Compare To Constant6 : simulink/Logic and Bit Operations/Compare To Constant  relop===  const=2  OutDataTypeStr=boolean
  Compare To Constant7 : simulink/Logic and Bit Operations/Compare To Constant  relop===  const=2  OutDataTypeStr=boolean
  Constant1 : Constant  Value=0
  Constant2 : Constant  Value=20
  Constant7 : Constant  Value=20
  Ego lane : simulink/Logic and Bit Operations/Compare To Constant  relop===  const=0  OutDataTypeStr=boolean
  Ego spd > 75 kph : simulink/Logic and Bit Operations/Compare To Constant  relop=>=  const=20.157  OutDataTypeStr=boolean
  Ego spd > set spd : RelationalOperator  Operator=>  OutDataTypeStr=boolean  RndMeth=Simplest  InputSameDT=off
  Gain1 : Gain  Gain=5  OutDataTypeStr=double
  Gain2 : Gain  Gain=2  OutDataTypeStr=double
  Gain5 : Gain  Gain=4  OutDataTypeStr=double
  Gain6 : Gain  Gain=2  OutDataTypeStr=double
  Left lane : simulink/Logic and Bit Operations/Compare To Constant  relop===  const=1  OutDataTypeStr=boolean
  Logical Operator{,6..8,10} (5 alike) : Logic  AllPortsSameDT=off  OutDataTypeStr=boolean
  Logical Operator{1..3,5,14} (5 alike) : Logic  Operator=OR  AllPortsSameDT=off  OutDataTypeStr=boolean
  Logical Operator4 : Logic  Operator=OR  Inputs=4  AllPortsSameDT=off  OutDataTypeStr=boolean
  Logical Operator9 : Logic  Inputs=4  AllPortsSameDT=off  OutDataTypeStr=boolean
  MinSpeed : Constant  Value=5.312
  Misuse : Stateflow chart  TreatAsAtomicUnit=on
  Not both : simulink/Logic and Bit Operations/Compare To Constant  relop=~=  const=3  OutDataTypeStr=boolean
  Override timeout : Stateflow chart  TreatAsAtomicUnit=on
  PA_State : Stateflow chart  TreatAsAtomicUnit=on
  Relational Operator : RelationalOperator  OutDataTypeStr=boolean  RndMeth=Simplest  InputSameDT=off
  Set spd > 150 kph : simulink/Logic and Bit Operations/Compare To Constant  relop=>  const=40.6111  OutDataTypeStr=boolean
  Speed too low : Logic  Operator=NOT  AllPortsSameDT=off  OutDataTypeStr=boolean
  Stop : simulink/Logic and Bit Operations/Compare To Constant  relop===  const=3  OutDataTypeStr=boolean
  Stop timeout : Stateflow chart  TreatAsAtomicUnit=on
  Terminator : Terminator
  Tgt spd < set spd : RelationalOperator  Operator=<=  OutDataTypeStr=boolean  RndMeth=Simplest  InputSameDT=off
  Tgt spd > 85 kph : simulink/Logic and Bit Operations/Compare To Constant  relop=>=  const=22.884  OutDataTypeStr=boolean
  Unit Delay7 : UnitDelay  SampleTime=-1  HasFrameUpgradeWarning=on
  SET_AccActvnOk : Outport
  SET_AccStopModOk : Outport  Port=2
  SET_VehTarDetd : Outport  Port=3
  SET_AccWarnForStatyTar : Outport  Port=4
  SET_UndertakePrevWarn : Outport  Port=5
  SET_DriveAwayInfoWarnReq : Outport  Port=6
  SET_AvlStsForLongAutDrv : Outport  Port=7
  SET_CnclWarnLgtForAutDrv : Outport  Port=8
  SET_AccSts : Outport  Port=9
  SET_SteerAsscCtrlActv : Outport  Port=10
  SET_SteerAutDrvActvnOk : Outport  Port=11
  SET_AvlStsForSteerSpprt : Outport  Port=12
  wires:
  GET_CrsCtrlFctSeld/1 -> ACC_State/2(CrsCtrlFctSeld)
  Logical Operator5/1 -> Logical Operator10/1, Speed too low/1
  Tgt spd < set spd/1 -> Logical Operator/1
  Logical Operator2/1 -> SET_AccStopModOk/1, SET_VehTarDetd/1
  Logical Operator/1 -> Logical Operator6/1, Logical Operator9/1
  Relational Operator/1 -> Logical Operator5/1
  Constant1/1 -> SET_AccWarnForStatyTar/1
  GET_SetSpeed/1 -> Set spd > 150 kph/1, Ego spd > set spd/2, Tgt spd < set spd/2
  GET_SpdTar/1 -> Tgt spd > 85 kph/1, ACC_State/1(SpdTar), Compare To Constant4/1, Tgt spd < set spd/1
  Logical Operator9/1 -> Logical Operator2/2, SET_UndertakePrevWarn/1
  GET_TgtLane/1 -> Ego lane/1, Left lane/1
  Override timeout/1(Timeout) -> CancelWarning/4(Ovrd)
  Constant7/1 -> Override timeout/2(Time)
  Ego spd > set spd/1 -> Logical Operator7/2
  Logical Operator7/1 -> Override timeout/1(Set)
  GET_EscEmgyStop/1 -> Compare To Constant3/1
  Stop timeout/1(Timeout) -> CancelWarning/3(Stop)
  GET_VehSpd/1 -> Ego spd > set spd/1, Ego spd > 75 kph/1, Relational Operator/1
  Tgt spd > 85 kph/1 -> Logical Operator9/3
  Ego spd > 75 kph/1 -> Logical Operator9/4
  Logical Operator6/1 -> Logical Operator2/1
  Ego lane/1 -> Logical Operator6/2
  Active/1 -> Logical Operator7/1, Logical Operator3/2, Logical Operator14/2
  DriverBrake/1 -> Logical Operator4/3
  Stop/1 -> Logical Operator14/1, Logical Operator8/2, Logical Operator3/1, Logical Operator5/2
  GET_CtrlFctActvReq/1 -> ACC_State/3(Activate)
  GET_CtrlFctDeactReq/1 -> Logical Operator4/2
  MinSpeed/1 -> Relational Operator/2
  Logical Operator4/1 -> ACC_State/4(Deactivate)
  Unit Delay7/1 -> Logical Operator4/1
  Compare To Constant3/1 -> Logical Operator4/4, Misuse/1(EmgStop)
  Set spd > 150 kph/1 -> Gain5/1
  Add/1 -> Compare To Constant5/1, Compare To Constant1/1, SET_AvlStsForSteerSpprt/1
  CancelWarning/2(AvlSts) -> Compare To Constant2/1, SET_AvlStsForLongAutDrv/1
  Speed too low/1 -> CancelWarning/1(LoSpd)
  Gain5/1 -> Add/3
  Gain6/1 -> Add/2
  Misuse/1(NoSteer) -> Gain6/1
  AvlStsPA/1 -> Add/4, Add/1
  Compare To Constant1/1 -> SET_SteerAutDrvActvnOk/1
  Logical Operator3/1 -> Logical Operator/2
  PA_State/1(State) -> SET_SteerAsscCtrlActv/1
  Logical Operator10/1 -> SET_AccActvnOk/1
  Compare To Constant2/1 -> Logical Operator10/2
  Logical Operator14/1 -> ACC inactive/1, CancelWarning/2(Active)
  CancelWarning/3(CnclWrn) -> SET_CnclWarnLgtForAutDrv/1
  CancelWarning/1(Cncl) -> Unit Delay7/1
  ACC_State/1(State) -> Active/1, Stop timeout/1(State), SET_AccSts/1, Stop/1
  Constant2/1 -> Stop timeout/2(Time)
  Compare To Constant4/1 -> Logical Operator8/1
  Logical Operator8/1 -> Gain2/1
  Gain2/1 -> SET_DriveAwayInfoWarnReq/1
  GET_SteerAutDrvActvReq/1 -> Compare To Constant6/1
  Compare To Constant5/1 -> PA_State/3(Unavailable)
  Logical Operator1/1 -> PA_State/2(Deactivate)
  GET_SteerAutDrvDeactReq/1 -> Compare To Constant7/1
  ACC inactive/1 -> Logical Operator1/1
  Compare To Constant6/1 -> PA_State/1(Activate)
  Compare To Constant7/1 -> Logical Operator1/2
  Left lane/1 -> Logical Operator9/2
  Not both/1 -> Gain1/1
  GET_LaneDetSts/1 -> Not both/1
  Gain1/1 -> Terminator/1

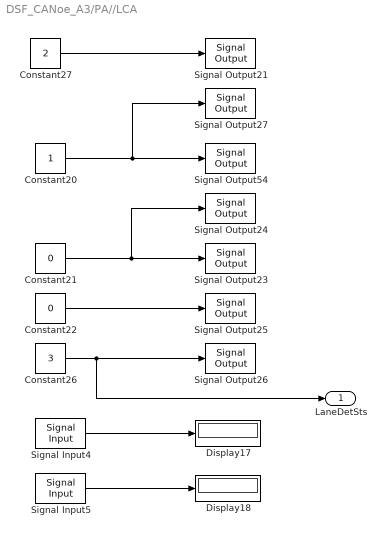
== system DSF_CANoe_A3/PA//LCA ==
  Constant20 : Constant  OutDataTypeStr=uint8
  Constant21 : Constant  Value=0
  Constant22 : Constant  Value=0
  Constant26 : Constant  Value=3  OutDataTypeStr=uint8
  Constant27 : Constant  Value=2  OutDataTypeStr=uint8
  Display17 : Display
  Display18 : Display
  Signal Input4 : canoelib/CANoe I//O/Signal Input  dbName=Backbone  nodeName=DIM  msgName=DIMBackBoneSignalIPdu02  sigName=SteerAutDrvActvReq  editSampleTime=0  rawValue=Default  dataType=Default  dataTypeDB=uint8  hasEncoding=off
      settings: AttributesFormatString=%<sigName>  SourceProductName=Vector CANoe
  Signal Input5 : canoelib/CANoe I//O/Signal Input  dbName=Backbone  nodeName=DIM  msgName=DIMBackBoneSignalIPdu02  sigName=SteerAutDrvDeactvnReq  editSampleTime=0  rawValue=Default  dataType=Default  dataTypeDB=uint8  hasEncoding=off
      settings: AttributesFormatString=%<sigName>  SourceProductName=Vector CANoe
  Signal Output21 : canoelib/CANoe I//O/Signal Output  dbName=Backbone  nodeName=ASDM  msgName=ASDMBackBoneSignalIPdu01  sigName=SteerStsForAutDrv  rawValue=Default  dataType=Default  dataTypeDB=uint8  hasEncoding=off
      settings: AttributesFormatString=%<sigName>  SourceProductName=Vector CANoe
  Signal Output23 : canoelib/CANoe I//O/Signal Output  dbName=Backbone  nodeName=ASDM  msgName=ASDMBackBoneSignalIPdu01  sigName=SteerOvrdWarnReqForAutDrv  rawValue=Default  dataType=Default  dataTypeDB=uint8  hasEncoding=off
      settings: AttributesFormatString=%<sigName>  SourceProductName=Vector CANoe
  Signal Output24 : canoelib/CANoe I//O/Signal Output  dbName=Backbone  nodeName=ASDM  msgName=ASDMBackBoneSignalIPdu02  sigName=SteerWarnReqForAutDrv  rawValue=Default  dataType=Default  dataTypeDB=uint8  hasEncoding=off
      settings: AttributesFormatString=%<sigName>  SourceProductName=Vector CANoe
  Signal Output25 : canoelib/CANoe I//O/Signal Output  dbName=Backbone  nodeName=ASDM  msgName=ASDMBackBoneSignalIPdu07  sigName=AvlStsForLatAutDrv  rawValue=Default  dataType=Default  dataTypeDB=uint8  hasEncoding=off
      settings: AttributesFormatString=%<sigName>  SourceProductName=Vector CANoe
  Signal Output26 : canoelib/CANoe I//O/Signal Output  dbName=Backbone  nodeName=ASDM  msgName=ASDMBackBoneSignalIPdu06  sigName=LaneDetnStsForAutDrv  rawValue=Default  dataType=Default  dataTypeDB=uint8  hasEncoding=off
      settings: AttributesFormatString=%<sigName>  SourceProductName=Vector CANoe
  Signal Output27 : canoelib/CANoe I//O/Signal Output  dbName=Backbone  nodeName=IHU  msgName=IHUBackBoneSignalIPdu08  sigName=VehSpdCtrlActvSts  rawValue=Default  dataType=Default  dataTypeDB=boolean  hasEncoding=off
      settings: AttributesFormatString=%<sigName>  SourceProductName=Vector CANoe
  Signal Output54 : canoelib/CANoe I//O/Signal Output  dbName=Backbone  nodeName=IHU  msgName=IHUBackBoneSignalIPdu04  sigName=SteerAssiActvForAutDrvSts  rawValue=Default  dataType=Default  dataTypeDB=boolean  hasEncoding=off
      settings: AttributesFormatString=%<sigName>  SourceProductName=Vector CANoe
  LaneDetSts : Outport
  wires:
  Constant27/1 -> Signal Output21/1
  Constant22/1 -> Signal Output25/1
  Constant21/1 -> Signal Output24/1, Signal Output23/1
  Constant26/1 -> LaneDetSts/1, Signal Output26/1
  Signal Input5/1 -> Display18/1
  Constant20/1 -> Signal Output54/1, Signal Output27/1
  Signal Input4/1 -> Display17/1

== system DSF_CANoe_A3/SCF ==
  Get_AccSts : Inport
  SCF : Constant
  SCF_SpdCtrlFctStst : Stateflow chart  TreatAsAtomicUnit=on
  SET_SpdCtrlFctSts : Outport
  wires:
  SCF/1 -> SCF_SpdCtrlFctStst/1(SCF_Status)
  Get_AccSts/1 -> SCF_SpdCtrlFctStst/2(GetAccSts)
  SCF_SpdCtrlFctStst/1(SetSpdCtrlFctSts) -> SET_SpdCtrlFctSts/1

== system DSF_CANoe_A3/SL ==
  Constant10 : Constant  Value=0  OutDataTypeStr=uint8
  Constant11 : Constant  Value=40/3.6  OutDataTypeStr=double
  Constant36 : Constant  OutDataTypeStr=uint8
  Constant4 : Constant  Value=0
  Constant6 : Constant  Value=0
  Signal Output33 : canoelib/CANoe I//O/Signal Output  dbName=Backbone  nodeName=VCU1  msgName=VDDMBackBoneSignalIPdu01  sigName=AdjSpdLimnWarn  rawValue=Default  dataType=Default  dataTypeDB=uint8  hasEncoding=off
      settings: AttributesFormatString=%<sigName>  SourceProductName=Vector CANoe
  Signal Output35 : canoelib/CANoe I//O/Signal Output  dbName=Backbone  nodeName=VCU1  msgName=VDDMBackBoneSignalIPdu01  sigName=AdjSpdLimnMsg  rawValue=Default  dataType=Default  dataTypeDB=uint8  hasEncoding=off
      settings: AttributesFormatString=%<sigName>  SourceProductName=Vector CANoe
  Signal Output40 : canoelib/CANoe I//O/Signal Output  dbName=Backbone  nodeName=CEM  msgName=CEMBackBoneSignalIpdu26  sigName=KeyRstrictdActvSpeedLimit  rawValue=Default  dataType=Default  dataTypeDB=uint16  hasEncoding=on
      settings: AttributesFormatString=%<sigName>  SourceProductName=Vector CANoe
  Signal Output41 : canoelib/CANoe I//O/Signal Output  dbName=Backbone  nodeName=CEM  msgName=CEMBackBoneSignalIpdu26  sigName=KeyRstrictdActvRestrictionStatus  rawValue=Default  dataType=Default  dataTypeDB=boolean  hasEncoding=off
      settings: AttributesFormatString=%<sigName>  SourceProductName=Vector CANoe
  Signal Output60 : canoelib/CANoe I//O/Signal Output  dbName=Backbone  nodeName=IHU  msgName=IHUBackBoneSignalIPdu03  sigName=RoadSgnInfoActvSts  rawValue=Default  dataType=Default  dataTypeDB=boolean  hasEncoding=off
      settings: AttributesFormatString=%<sigName>  SourceProductName=Vector CANoe
  KeySpdLim : Outport
  KeySts : Outport  Port=2
  wires:
  Constant4/1 -> Signal Output33/1
  Constant11/1 -> KeySpdLim/1, Signal Output40/1
  Constant6/1 -> Signal Output35/1
  Constant10/1 -> KeySts/1, Signal Output41/1
  Constant36/1 -> Signal Output60/1

== system DSF_CANoe_A3/SL model ==
  GET_DrvrCrsCtrlFctSeld : Inport
  GET_DrvrCrsCtrlFctActvReq : Inport  Port=2
  GET_DrvrCrsCtrlFctDeactvnReq : Inport  Port=3
  GET_CrsCtrlOvrdn : Inport  Port=4
  Constant3 : Constant  OutDataTypeStr=uint8
  SL_State : Stateflow chart  TreatAsAtomicUnit=on
  SET_AdjSpdLimnSts : Outport
  SET_AdjSpdLimnActvOk : Outport  Port=2
  wires:
  GET_DrvrCrsCtrlFctActvReq/1 -> SL_State/2(Activate)
  GET_DrvrCrsCtrlFctSeld/1 -> SL_State/1(CrsCtrlFctSeld)
  GET_DrvrCrsCtrlFctDeactvnReq/1 -> SL_State/3(Deactivate)
  SL_State/1(State) -> SET_AdjSpdLimnSts/1
  GET_CrsCtrlOvrdn/1 -> SL_State/4(CrsCtrlOvrdn)
  Constant3/1 -> SET_AdjSpdLimnActvOk/1
